simulink model "PID_Dinamic_Kinematic"  (R2020b)
settings: Solver=ode4  StartTime=0.0  StopTime=30  FixedStep=0.01  RelTol=1e-3
values from neighbouring files (symbols this model uses):
  a = 0    [Robot_Parameters.m]
  b = 0.2    [Robot_Parameters.m]
  I = 0.08    [Robot_Parameters.m]
  Ke = 0.03    [Robot_Parameters.m]
  Kt = 0.001    [Robot_Parameters.m]
  L = 0.01    [Robot_Parameters.m]
  m = 1.733    [Robot_Parameters.m]
  N = 30    [Robot_Parameters.m]
  r = 0.0425    [Robot_Parameters.m]
  R = 0.7    [Robot_Parameters.m]
libraries: pid_lib x2, simulink x1
settings Model: OrderedModelArguments=off  Creator=dell  LastModifiedBy=dell

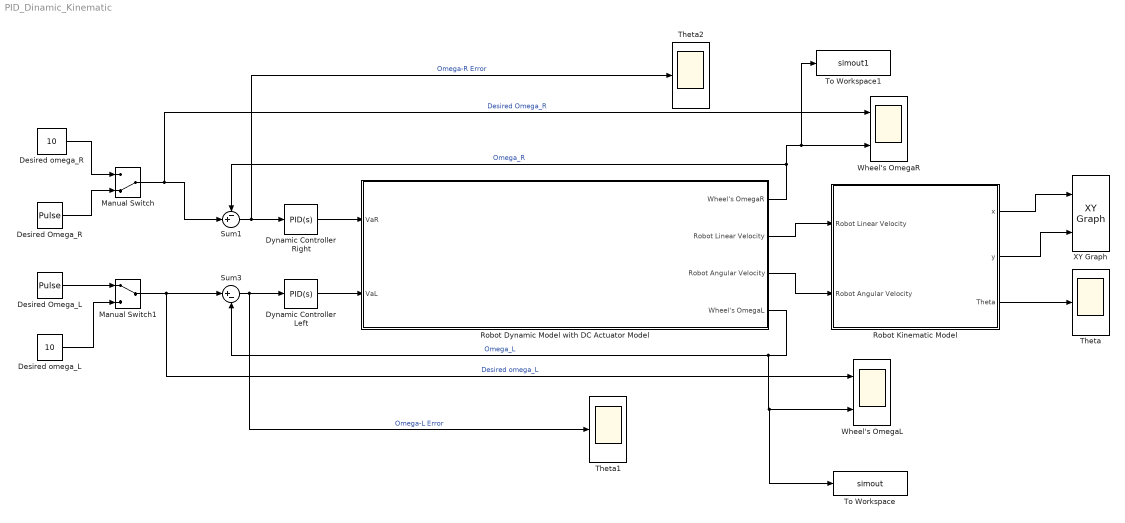
== system PID_Dinamic_Kinematic ==
  Desired Omega_L : DiscretePulseGenerator  PulseType=Time based  Amplitude=10  Period=10  PulseWidth=50
  Desired Omega_R : DiscretePulseGenerator  PulseType=Time based  Amplitude=10  Period=10  PulseWidth=50
  Desired omega_L : Constant  Value=10
  Desired omega_R : Constant  Value=10
  Dynamic Controller Left : pid_lib/PID Controller  Controller=PID  Form=Parallel  TimeDomain=Continuous-time  UseExternalTs=off  SampleTime=-1  IntegratorMethod=Forward Euler  FilterMethod=Forward Euler  ControllerParametersSource=internal  P=0.75291038869307  I=8.52783510111841  D=-0.0138279489870919  UseFilter=on  N=14.2847240550013  TunerSelectOption=Transfer Function Based (PID Tuner App)  InitialConditionSource=internal  InitialConditionForIntegrator=0  InitialConditionForFilter=0  DifferentiatorICPrevScaledInput=0  ExternalReset=none  TrackingMode=off  Kt=1  LimitOutput=off  SatLimitsSource=internal  UpperSaturationLimit=inf  LowerSaturationLimit=-inf  LinearizeAsGain=on  AntiWindupMode=none  Kb=1  POutMin=[]  POutMax=[]  IOutMin=[]  IOutMax=[]  DOutMin=[]  DOutMax=[]  NOutMin=[]  NOutMax=[]  SumOutMin=[]  SumOutMax=[]  SaturationOutMin=[]  SaturationOutMax=[]  PParamMin=[]  PParamMax=[]  IParamMin=[]  IParamMax=[]  DParamMin=[]  DParamMax=[]  NParamMin=[]  NParamMax=[]  KbParamMin=[]  KbParamMax=[]  KtParamMin=[]  KtParamMax=[]  KbOutMin=[]  KbOutMax=[]  KtOutMin=[]  KtOutMax=[]  IntegratorOutMin=[]  IntegratorOutMax=[]  FilterOutMin=[]  FilterOutMax=[]  SumI1OutMin=[]  SumI1OutMax=[]  SumI2OutMin=[]  SumI2OutMax=[]  SumI3OutMin=[]  SumI3OutMax=[]  SumI4OutMin=[]  SumI4OutMax=[]  SumDOutMin=[]  SumDOutMax=[]  DifferentiatorOutMin=[]  DifferentiatorOutMax=[]  FilterDiffOutCoefMin=[]  FilterDiffOutCoefMax=[]  ReciprocalOutMin=[]  ReciprocalOutMax=[]  SumDenOutMin=[]  SumDenOutMax=[]  SumNumOutMin=[]  SumNumOutMax=[]  DivideOutMin=[]  DivideOutMax=[]  UdiffTsProdOutMin=[]  UdiffTsProdOutMax=[]  NTsProdOutMin=[]  NTsProdOutMax=[]  UintegralTsProdOutMin=[]  UintegralTsProdOutMax=[]  UngainTsProdOutMin=[]  UngainTsProdOutMax=[]  IntegratorContinuousStateAttributes=''  IntegratorStateMustResolveToSignalObject=off  IntegratorRTWStateStorageClass=Auto  FilterContinuousStateAttributes=''  FilterStateMustResolveToSignalObject=off  FilterRTWStateStorageClass=Auto  ParallelPVariant=InternalParameters  IdealPVariant=Disabled  IVariant=InternalParameters  DVariant=InternalParameters  IntegratorVariant=Continuous  SatVariant=Disabled  AWVariant=Passthrough  PCopyVariant=Disabled  TRVariant=Disabled  FdbkBlocksVariant=Forward  IdealPFdbkVariant=Disabled  SatFdbkVariant=Disabled  DerivativeFilterVariant=ContFilter  NVariant=InternalParameters  NCopyVariant=Disabled  FilterICVariant=InternalICsFilter  IntegratorICVariant=InternalICs  ExternalResetVariant=Disabled  TRSumVariant=Passthrough  SumFdbkVariant=Disabled  SumVariant=Sum_PID  TsampFilterVariant=InternalTs  TsampNgainVariant=Passthrough  TsampIntegralVariant=Passthrough  ExternalSaturationOutDataTypeStr=Inherit: Same as second input
  Dynamic Controller Right : pid_lib/PID Controller  Controller=PID  Form=Parallel  TimeDomain=Continuous-time  UseExternalTs=off  SampleTime=-1  IntegratorMethod=Forward Euler  FilterMethod=Forward Euler  ControllerParametersSource=internal  P=0.926055377132756  I=9.27563715391367  D=-0.025  UseFilter=on  N=20.0890041410903  TunerSelectOption=Transfer Function Based (PID Tuner App)  ZeroCross=off  InitialConditionSource=internal  InitialConditionForIntegrator=0  InitialConditionForFilter=0  DifferentiatorICPrevScaledInput=0  ExternalReset=none  TrackingMode=off  Kt=1  LimitOutput=off  SatLimitsSource=internal  UpperSaturationLimit=inf  LowerSaturationLimit=-inf  LinearizeAsGain=on  AntiWindupMode=none  Kb=1  POutMin=[]  POutMax=[]  IOutMin=[]  IOutMax=[]  DOutMin=[]  DOutMax=[]  NOutMin=[]  NOutMax=[]  SumOutMin=[]  SumOutMax=[]  SaturationOutMin=[]  SaturationOutMax=[]  PParamMin=[]  PParamMax=[]  IParamMin=[]  IParamMax=[]  DParamMin=[]  DParamMax=[]  NParamMin=[]  NParamMax=[]  KbParamMin=[]  KbParamMax=[]  KtParamMin=[]  KtParamMax=[]  KbOutMin=[]  KbOutMax=[]  KtOutMin=[]  KtOutMax=[]  IntegratorOutMin=[]  IntegratorOutMax=[]  FilterOutMin=[]  FilterOutMax=[]  SumI1OutMin=[]  SumI1OutMax=[]  SumI2OutMin=[]  SumI2OutMax=[]  SumI3OutMin=[]  SumI3OutMax=[]  SumI4OutMin=[]  SumI4OutMax=[]  SumDOutMin=[]  SumDOutMax=[]  DifferentiatorOutMin=[]  DifferentiatorOutMax=[]  FilterDiffOutCoefMin=[]  FilterDiffOutCoefMax=[]  ReciprocalOutMin=[]  ReciprocalOutMax=[]  SumDenOutMin=[]  SumDenOutMax=[]  SumNumOutMin=[]  SumNumOutMax=[]  DivideOutMin=[]  DivideOutMax=[]  UdiffTsProdOutMin=[]  UdiffTsProdOutMax=[]  NTsProdOutMin=[]  NTsProdOutMax=[]  UintegralTsProdOutMin=[]  UintegralTsProdOutMax=[]  UngainTsProdOutMin=[]  UngainTsProdOutMax=[]  IntegratorContinuousStateAttributes=''  IntegratorStateMustResolveToSignalObject=off  IntegratorRTWStateStorageClass=Auto  FilterContinuousStateAttributes=''  FilterStateMustResolveToSignalObject=off  FilterRTWStateStorageClass=Auto  ParallelPVariant=InternalParameters  IdealPVariant=Disabled  IVariant=InternalParameters  DVariant=InternalParameters  IntegratorVariant=Continuous  SatVariant=Disabled  AWVariant=Passthrough  PCopyVariant=Disabled  TRVariant=Disabled  FdbkBlocksVariant=Forward  IdealPFdbkVariant=Disabled  SatFdbkVariant=Disabled  DerivativeFilterVariant=ContFilter  NVariant=InternalParameters  NCopyVariant=Disabled  FilterICVariant=InternalICsFilter  IntegratorICVariant=InternalICs  ExternalResetVariant=Disabled  TRSumVariant=Passthrough  SumFdbkVariant=Disabled  SumVariant=Sum_PID  TsampFilterVariant=InternalTs  TsampNgainVariant=Passthrough  TsampIntegralVariant=Passthrough  ExternalSaturationOutDataTypeStr=Inherit: Same as second input
  Manual Switch : ManualSwitch  CurrentSetting=0
  Manual Switch1 : ManualSwitch
  Robot Dynamic Model with DC Actuator Model : Subsystem
  Robot Kinematic Model : Subsystem
  Sum1 : Sum  Inputs=-+|
  Sum3 : Sum  Inputs=|+-
  Theta : Scope
  Theta1 : Scope
  Theta2 : Scope
  To Workspace : ToWorkspace  VariableName=simout  SaveFormat=Timeseries  SampleTime=-1
  To Workspace1 : ToWorkspace  VariableName=simout1  SaveFormat=Timeseries  SampleTime=-1
  Wheel's OmegaL : Scope  NumInputPorts=2
  Wheel's OmegaR : Scope  NumInputPorts=2
  XY Graph : simulink/Sinks/XY Graph  xmin=-2.5  xmax=2.5  ymin=-0.5  ymax=5  st=-1
  wires:
  Sum1/1 -> Theta2/1, Dynamic Controller Right/1  "Omega-R Error"
  Sum3/1 -> Theta1/1, Dynamic Controller Left/1  "Omega-L Error"
  Robot Kinematic Model/1(x) -> XY Graph/1
  Robot Kinematic Model/2(y) -> XY Graph/2
  Robot Kinematic Model/3(Theta) -> Theta/1
  Robot Dynamic Model with DC Actuator Model/2(Robot Linear Velocity) -> Robot Kinematic Model/1(Robot Linear Velocity)
  Robot Dynamic Model with DC Actuator Model/3(Robot Angular Velocity) -> Robot Kinematic Model/2(Robot Angular Velocity)
  Dynamic Controller Right/1 -> Robot Dynamic Model with DC Actuator Model/1(VaR)
  Dynamic Controller Left/1 -> Robot Dynamic Model with DC Actuator Model/2(VaL)
  Robot Dynamic Model with DC Actuator Model/1(Wheel's OmegaR) -> Sum1/1, To Workspace1/1, Wheel's OmegaR/2  "Omega_R"
  Robot Dynamic Model with DC Actuator Model/4(Wheel's OmegaL) -> To Workspace/1, Wheel's OmegaL/2, Sum3/2  "Omega_L"
  Desired omega_L/1 -> Manual Switch1/2
  Manual Switch/1 -> Wheel's OmegaR/1, Sum1/2  "Desired Omega_R"
  Desired omega_R/1 -> Manual Switch/1
  Desired Omega_R/1 -> Manual Switch/2
  Manual Switch1/1 -> Wheel's OmegaL/1, Sum3/1  "Desired omega_L"
  Desired Omega_L/1 -> Manual Switch1/1

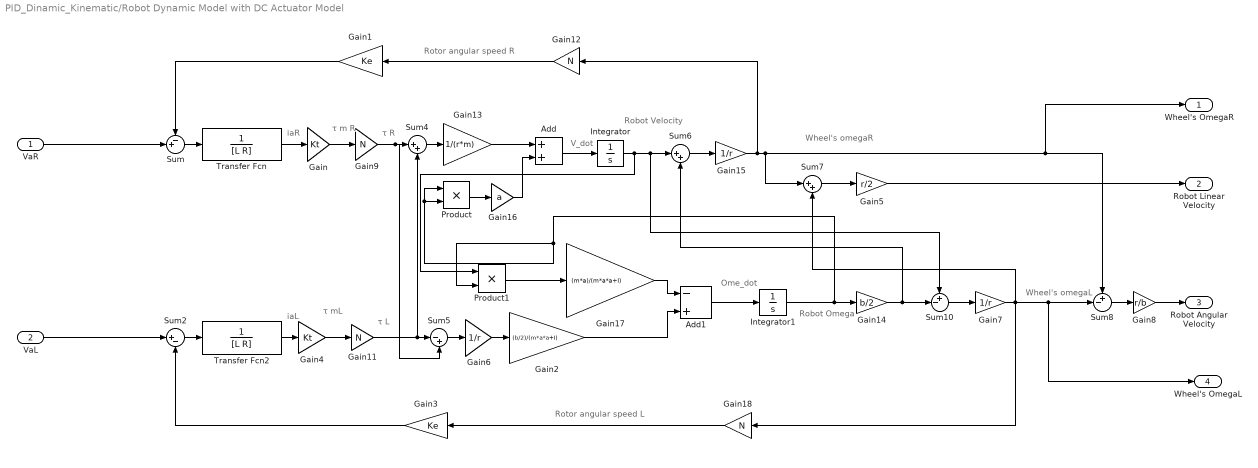
== system PID_Dinamic_Kinematic/Robot Dynamic Model with DC Actuator Model ==
  note: Rotor angular speed R
  note: Robot Velocity
  note: V_dot
  note: Robot Omega
  note: Ome_dot
  note: τ R
  note: τ m R
  note: iaR
  note: iaL
  note: τ mL
  note: τ L
  note: Rotor angular speed L
  note: Wheel's omegaR
  note: Wheel's omegaL
  VaR : Inport
  VaL : Inport  Port=2
  Add : Sum
  Add1 : Sum  Inputs=-+
  Gain : Gain  Gain=Kt
  Gain1 : Gain  Gain=Ke
  Gain{9,11..12,18} (4 alike) : Gain  Gain=N
  Gain13 : Gain  Gain=1/(r*m)
  Gain14 : Gain  Gain=b/2
  Gain15 : Gain  Gain=1/r
  Gain16 : Gain  Gain=a
  Gain17 : Gain  Gain=(m*a)/(m*a*a+I)
  Gain2 : Gain  Gain=(b/2)/(m*a*a+I)
  Gain3 : Gain  Gain=Ke
  Gain4 : Gain  Gain=Kt
  Gain5 : Gain  Gain=r/2
  Gain6 : Gain  Gain=1/r
  Gain7 : Gain  Gain=1/r
  Gain8 : Gain  Gain=r/b
  Integrator : Integrator
  Integrator1 : Integrator
  Product : Product
  Product1 : Product
  Sum : Sum  Inputs=-+|
  Sum10 : Sum  Inputs=+-|
  Sum2 : Sum  Inputs=|+-
  Sum4 : Sum  Inputs=|++
  Sum5 : Sum  Inputs=|-+
  Sum6 : Sum  Inputs=|++
  Sum7 : Sum  Inputs=|++
  Sum8 : Sum  Inputs=+-|
  Transfer Fcn : TransferFcn  Denominator=[L R]
  Transfer Fcn2 : TransferFcn  Denominator=[L R]
  Wheel's OmegaR : Outport
  Robot Linear Velocity : Outport  Port=2
  Robot Angular Velocity : Outport  Port=3
  Wheel's OmegaL : Outport  Port=4
  wires:
  Gain8/1 -> Robot Angular Velocity/1
  Gain5/1 -> Robot Linear Velocity/1
  Integrator/1 -> Sum6/1, Sum10/1, Product1/1
  Gain2/1 -> Add1/2
  Gain4/1 -> Gain11/1
  Sum6/1 -> Gain15/1
  Gain14/1 -> Sum10/2, Sum6/2
  Gain1/1 -> Sum/1
  Gain15/1 -> Gain12/1, Wheel's OmegaR/1, Sum8/1, Sum7/1
  Sum7/1 -> Gain5/1
  Gain6/1 -> Gain2/1
  Integrator1/1 -> Gain14/1, Product/2, Product/1, Product1/2
  Sum10/1 -> Gain7/1
  Product1/1 -> Gain17/1
  Transfer Fcn2/1 -> Gain4/1
  Sum/1 -> Transfer Fcn/1
  Gain17/1 -> Add1/1
  Add/1 -> Integrator/1
  Add1/1 -> Integrator1/1
  Gain12/1 -> Gain1/1
  Gain7/1 -> Wheel's OmegaL/1, Sum8/2, Sum7/2, Gain18/1
  Product/1 -> Gain16/1
  Gain9/1 -> Sum4/1, Sum5/2
  Gain/1 -> Gain9/1
  Gain11/1 -> Sum5/1, Sum4/2
  Gain16/1 -> Add/2
  Sum8/1 -> Gain8/1
  Gain18/1 -> Gain3/1
  Sum2/1 -> Transfer Fcn2/1
  Gain3/1 -> Sum2/2
  VaL/1 -> Sum2/1
  Transfer Fcn/1 -> Gain/1
  Gain13/1 -> Add/1
  Sum4/1 -> Gain13/1
  Sum5/1 -> Gain6/1
  VaR/1 -> Sum/2

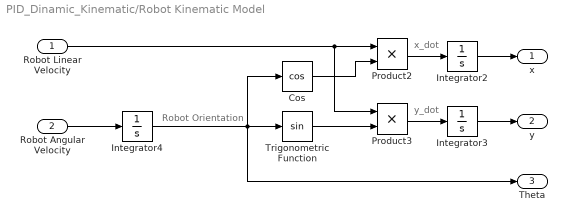
== system PID_Dinamic_Kinematic/Robot Kinematic Model ==
  note: x_dot
  note: Robot Orientation
  note: y_dot
  Robot Linear Velocity : Inport
  Robot Angular Velocity : Inport  Port=2
  Cos : Trigonometry  Operator=cos
  Integrator2 : Integrator
  Integrator3 : Integrator
  Integrator4 : Integrator
  Product2 : Product
  Product3 : Product
  Trigonometric Function : Trigonometry
  x : Outport
  y : Outport  Port=2
  Theta : Outport  Port=3
  wires:
  Trigonometric Function/1 -> Product3/2
  Cos/1 -> Product2/2
  Robot Linear Velocity/1 -> Product2/1, Product3/1
  Integrator4/1 -> Cos/1, Theta/1, Trigonometric Function/1
  Integrator2/1 -> x/1
  Product3/1 -> Integrator3/1
  Product2/1 -> Integrator2/1
  Integrator3/1 -> y/1
  Robot Angular Velocity/1 -> Integrator4/1
